simulink model "Sim_LQG_LTR_fenom"  (R2015a)
settings: Solver=ode45  StartTime=0.0  StopTime=t_run  RelTol=1e-3
values from neighbouring files (symbols this model uses):
  A = [-0.235284      0          0        0 ... (first row only)    [LQG_LTR_ident.m]    (also in Model.m = [-1/T(1) 0 area_maior(3)/(area_maior(1)*T(3)) 0 ; 0 -1/T(2) )
  A1 = 254.469    [LQG_LTR_fen.m]    (also in LQG_LTR_ident.m; LQG_LTR_pheno.m)
  a1 = 0.466    [LQG_LTR_fen.m]    (also in LQG_LTR_ident.m; LQG_LTR_pheno.m)
  a2 = 0.466    [LQG_LTR_fen.m]    (also in LQG_LTR_ident.m; LQG_LTR_pheno.m)
  A2 = 254.469    [LQG_LTR_fen.m]    (also in LQG_LTR_ident.m; LQG_LTR_pheno.m)
  a3 = 0.3421    [LQG_LTR_fen.m]    (also in LQG_LTR_ident.m; LQG_LTR_pheno.m)
  A3 = 254.469    [LQG_LTR_fen.m]    (also in LQG_LTR_ident.m; LQG_LTR_pheno.m)
  a4 = 0.3421    [LQG_LTR_fen.m]    (also in LQG_LTR_ident.m; LQG_LTR_pheno.m)
  A4 = 254.469    [LQG_LTR_fen.m]    (also in LQG_LTR_ident.m; LQG_LTR_pheno.m)
  B = [ -0.181039          0.00549506 ... (first row only)    [LQG_LTR_ident.m]    (also in Model.m = [gamma(1)*k(1)/area_maior(1) 0; 0 gamma(2)*k(2)/area_maior(2)
  C = [-0.498597  -0.23744    6.8883   -5.76097 ... (first row only)    [LQG_LTR_ident.m]    (also in Model.m = [kc 0 0 0; 0 kc 0 0])
  D = [0 0 ... (first row only)    [LQG_LTR_ident.m]    (also in Model.m = zeros(2))
  g = 980    [LQG_LTR_fen.m]    (also in LQG_LTR_ident.m; LQG_LTR_pheno.m; Model.m = 981)
  gamma_1 = 0.6    [LQG_LTR_fen.m]    (also in LQG_LTR_ident.m; LQG_LTR_pheno.m = 0.75)
  gamma_2 = 0.6    [LQG_LTR_fen.m]    (also in LQG_LTR_ident.m; LQG_LTR_pheno.m = 0.74)
  hinicial = [9 7 0 0]    [LQG_LTR_fen.m]    (also in LQG_LTR_ident.m; LQG_LTR_pheno.m; Model.m = [hi1 hi2 0 0])
  k1 = 18    [LQG_LTR_fen.m]    (also in LQG_LTR_ident.m; LQG_LTR_pheno.m = 12)
  k2 = 18    [LQG_LTR_fen.m]    (also in LQG_LTR_ident.m; LQG_LTR_pheno.m = 12)
  Kf = minreal(ss(Kc,'minimal'),1e-4)    [LQG_LTR_fen.m]    (also in LQG_LTR_ident.m; LQG_LTR_pheno.m)
  Ts = 0.1    [LQG_LTR_fen.m]    (also in LQG_LTR_ident.m; LQG_LTR_pheno.m)
settings Model: Creator=pcosta  LastModifiedBy=plinio

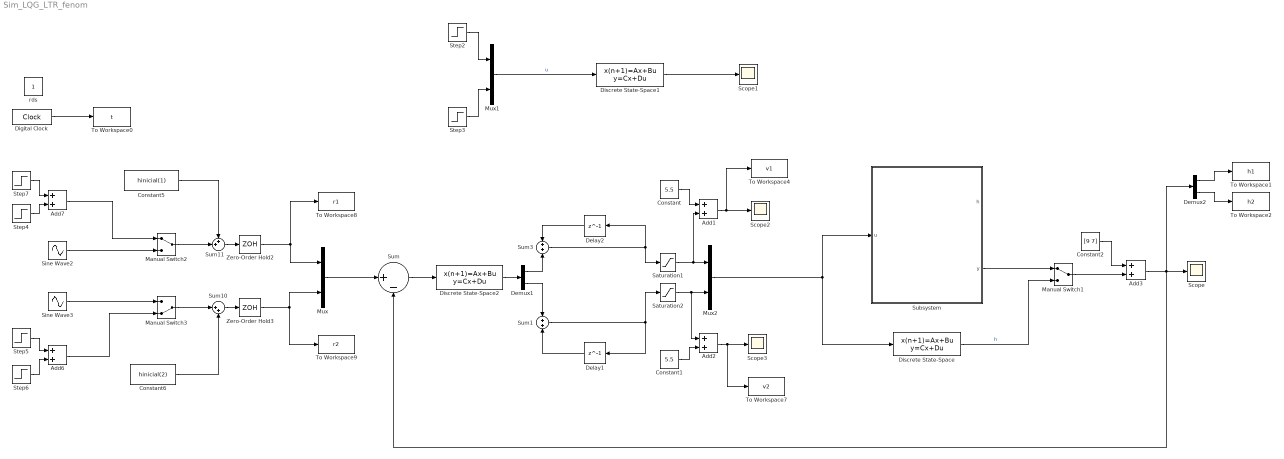
== system Sim_LQG_LTR_fenom ==
  Add{1..3,6..7} (5 alike) : Sum
  Constant : Constant  Value=5.5
  Constant1 : Constant  Value=5.5
  Constant2 : Constant  Value=[9 7]
  Constant5 : Constant  Value=hinicial(1)
  Constant6 : Constant  Value=hinicial(2)
  Delay1 : Delay  DelayLength=1  InitialCondition=0  SampleTime=Ts
  Delay2 : Delay  DelayLength=1  InitialCondition=0  SampleTime=Ts
  Demux1 : Demux  Outputs=2
  Demux2 : Demux  Outputs=2
  Digital Clock : DigitalClock  SampleTime=Ts
  Discrete State-Space : DiscreteStateSpace  A=A  B=B  C=C  D=D  SampleTime=Ts
  Discrete State-Space1 : DiscreteStateSpace  A=A  B=B  C=C  D=D  SampleTime=Ts
  Discrete State-Space2 : DiscreteStateSpace  A=Kf.a  B=Kf.b  C=Kf.c  D=Kf.d
  Manual Switch1 : ManualSwitch
  Manual Switch2 : ManualSwitch
  Manual Switch3 : ManualSwitch  CurrentSetting=0
  Mux : Mux  Inputs=2
  Mux1 : Mux  Inputs=2
  Mux2 : Mux  Inputs=2
  Saturation1 : Saturate  UpperLimit=4.5  LowerLimit=-5.5
  Saturation2 : Saturate  UpperLimit=4.5  LowerLimit=-5.5
  Scope{,1..3} (4 alike) : Scope
      Scope2 settings: SaveName=ScopeData2
      Scope3 settings: SaveName=ScopeData3
  Sine Wave2 : Sin  Frequency=0.1  SampleTime=0
  Sine Wave3 : Sin  Frequency=0.1  Phase=pi/2  SampleTime=0
  Step2 : Step  Time=0  After=5.5  SampleTime=Ts
  Step3 : Step  Time=0  After=5.5  SampleTime=Ts
  Step4 : Step  Time=400  After=-3  SampleTime=0  ZeroCross=off
  Step5 : Step  Time=200  After=3  SampleTime=0  ZeroCross=off
  Step6 : Step  Time=600  After=-3  SampleTime=0  ZeroCross=off
  Step7 : Step  Time=10  After=3  SampleTime=0  ZeroCross=off
  Subsystem : Subsystem
      mask Display: image(imread('/home/plinio/Dropbox/Mestrado_Plinio/Mestrado/Trabalho no Latex/Figuras/QuadTank.png'))
  Sum : Sum  Inputs=|+-
  Sum1 : Sum
  Sum10 : Sum  Inputs=|++
  Sum11 : Sum  Inputs=++|
  Sum3 : Sum
  To Workspace0 : ToWorkspace  VariableName=t  SampleTime=-1
  To Workspace1 : ToWorkspace  VariableName=h1  SampleTime=-1
  To Workspace2 : ToWorkspace  VariableName=h2  SampleTime=-1
  To Workspace4 : ToWorkspace  VariableName=v1  SampleTime=-1
  To Workspace7 : ToWorkspace  VariableName=v2  SampleTime=-1
  To Workspace8 : ToWorkspace  VariableName=r1  SampleTime=-1
  To Workspace9 : ToWorkspace  VariableName=r2  SampleTime=-1
  Zero-Order Hold2 : ZeroOrderHold  SampleTime=Ts
  Zero-Order Hold3 : ZeroOrderHold  SampleTime=Ts
  rds : Constant  IOType=siggen
  wires:
  Mux/1 -> Sum/1
  Discrete State-Space1/1 -> Scope1/1
  Mux1/1 -> Discrete State-Space1/1  "u"
  Step2/1 -> Mux1/1
  Step3/1 -> Mux1/2
  Discrete State-Space2/1 -> Demux1/1
  Sum3/1 -> Saturation1/1, Delay2/1
  Delay2/1 -> Sum3/1
  Sum1/1 -> Saturation2/1, Delay1/1
  Demux1/1 -> Sum3/2
  Saturation2/1 -> Mux2/2, Add2/1
  Saturation1/1 -> Add1/2, Mux2/1
  Constant/1 -> Add1/1
  Add1/1 -> To Workspace4/1, Scope2/1
  Add2/1 -> Scope3/1, To Workspace7/1
  Constant1/1 -> Add2/2
  Constant2/1 -> Add3/1
  Add3/1 -> Sum/2, Demux2/1, Scope/1
  Demux2/1 -> To Workspace1/1
  Demux2/2 -> To Workspace2/1
  Digital Clock/1 -> To Workspace0/1
  Sum/1 -> Discrete State-Space2/1
  Demux1/2 -> Sum1/1
  Delay1/1 -> Sum1/2
  Sum10/1 -> Zero-Order Hold3/1
  Constant6/1 -> Sum10/2
  Step4/1 -> Add7/2
  Step7/1 -> Add7/1
  Constant5/1 -> Sum11/1
  Step5/1 -> Add6/1
  Step6/1 -> Add6/2
  Sum11/1 -> Zero-Order Hold2/1
  Zero-Order Hold2/1 -> Mux/1, To Workspace8/1
  Add7/1 -> Manual Switch2/1
  Sine Wave2/1 -> Manual Switch2/2
  Sine Wave3/1 -> Manual Switch3/1
  Add6/1 -> Manual Switch3/2
  Manual Switch3/1 -> Sum10/1
  Manual Switch2/1 -> Sum11/2
  Zero-Order Hold3/1 -> Mux/2, To Workspace9/1
  Discrete State-Space/1 -> Manual Switch1/2  "h"
  Manual Switch1/1 -> Add3/2
  Mux2/1 -> Discrete State-Space/1, Subsystem/1(u)
  Subsystem/2(y) -> Manual Switch1/1

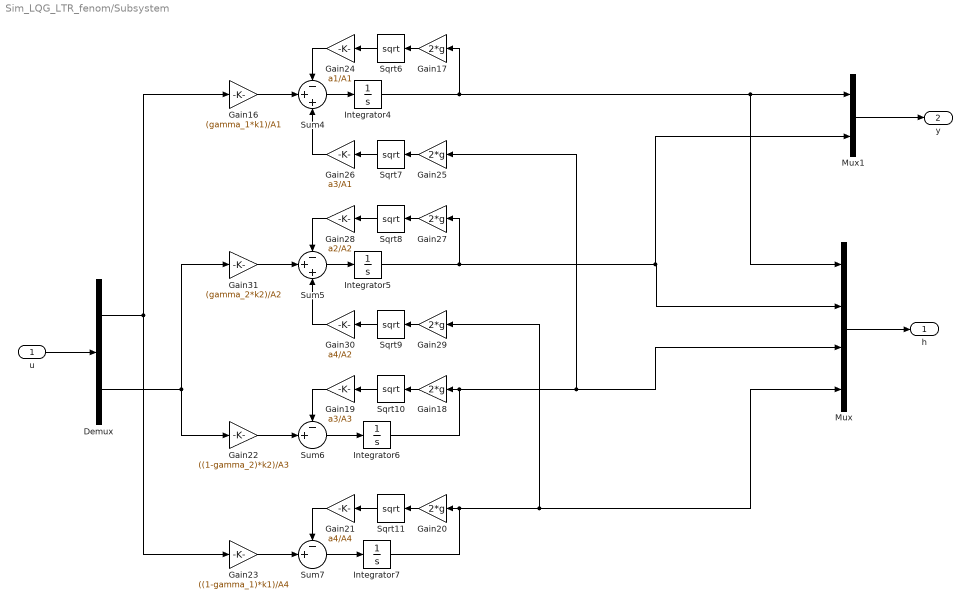
== system Sim_LQG_LTR_fenom/Subsystem ==
  u : Inport
  Demux : Demux  Outputs=2
  Gain16 : Gain  Gain=(gamma_1*k1)/A1
  Gain{17..18,20,25,27,29} (6 alike) : Gain  Gain=2*g
  Gain19 : Gain  Gain=a3/A3
  Gain21 : Gain  Gain=a4/A4
  Gain22 : Gain  Gain=((1-gamma_2)*k2)/A3
  Gain23 : Gain  Gain=((1-gamma_1)*k1)/A4
  Gain24 : Gain  Gain=a1/A1
  Gain26 : Gain  Gain=a3/A1
  Gain28 : Gain  Gain=a2/A2
  Gain30 : Gain  Gain=a4/A2
  Gain31 : Gain  Gain=(gamma_2*k2)/A2
  Integrator{4..7} (4 alike) : Integrator
  Mux : Mux
  Mux1 : Mux  Inputs=2
  Sqrt{6..11} (6 alike) : Sqrt  SaturateOnIntegerOverflow=on
  Sum4 : Sum  Inputs=-++
  Sum5 : Sum  Inputs=-++
  Sum6 : Sum  Inputs=-+|
  Sum7 : Sum  Inputs=-+|
  h : Outport
  y : Outport  Port=2
  wires:
  Gain30/1 -> Sum5/3
  Integrator7/1 -> Gain20/1, Gain29/1, Mux/4
  Sum7/1 -> Integrator7/1
  Gain23/1 -> Sum7/2
  Sum5/1 -> Integrator5/1
  Gain24/1 -> Sum4/1
  Sqrt6/1 -> Gain24/1
  Sum4/1 -> Integrator4/1
  Gain31/1 -> Sum5/2
  Gain27/1 -> Sqrt8/1
  Sqrt11/1 -> Gain21/1
  Gain18/1 -> Sqrt10/1
  Integrator5/1 -> Gain27/1, Mux/2, Mux1/2
  Sqrt9/1 -> Gain30/1
  Sqrt10/1 -> Gain19/1
  Gain16/1 -> Sum4/2
  Gain21/1 -> Sum7/1
  Sqrt8/1 -> Gain28/1
  Integrator4/1 -> Mux/1, Mux1/1, Gain17/1
  Gain26/1 -> Sum4/3
  Gain19/1 -> Sum6/1
  Gain22/1 -> Sum6/2
  Gain20/1 -> Sqrt11/1
  Sqrt7/1 -> Gain26/1
  Gain29/1 -> Sqrt9/1
  Sum6/1 -> Integrator6/1
  Gain17/1 -> Sqrt6/1
  Gain28/1 -> Sum5/1
  Integrator6/1 -> Gain18/1, Gain25/1, Mux/3
  Gain25/1 -> Sqrt7/1
  u/1 -> Demux/1
  Demux/2 -> Gain22/1, Gain31/1
  Demux/1 -> Gain23/1, Gain16/1
  Mux1/1 -> y/1
  Mux/1 -> h/1
